simulink model "Psk"  (Simulink 8.9)
settings: Solver=ode45  StartTime=0.0  StopTime=100  RelTol=1e-3  EnableMultiTasking=on
libraries: commrandsrc2 x1, dsparch4 x1
settings Model: Creator=Abhishek  LastModifiedBy=JBlanco
settings DataIOCC: SignalLoggingSaveFormat=Dataset
settings DebuggingCC: SolverPrmCheckMsg=warning  FcnCallInpInsideContextMsg=error
settings GRTTargetCC: CombineOutputUpdateFcns=on  GRTInterface=off

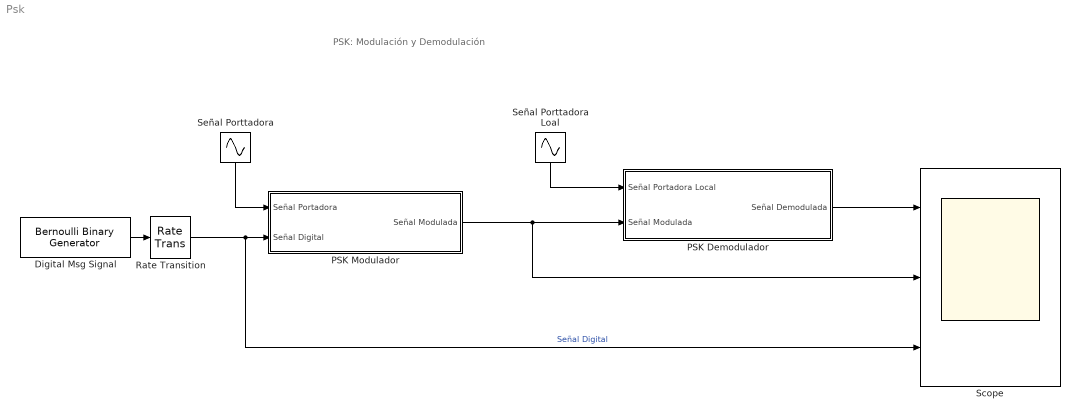
== system Psk ==
  note: PSK: Modulación y Demodulación
  Digital Msg Signal : commrandsrc2/Bernoulli Binary Generator  P=0.5  seed=61  Ts=5  frameBased=off  sampPerFrame=1  orient=off  outDataType=double  mask(Bernoulli Binary Generator){}
      mask Display:
      | % This is a new mask on top of the base mask.
      | % Use "View base mask" link below to see the base mask.
      | disp('Digital Data Gen.')
  PSK Demodulador : Subsystem
  PSK Modulador : Subsystem
  Rate Transition : RateTransition  OutPortSampleTime=1/2000
  Scope : Scope  NumInputPorts=3
  "Señal Porttadora " : Sin  Amplitude=5  Frequency=10*2*pi  Samples=50  SampleTime=1/2000
  Señal Porttadora Loal : Sin  Amplitude=5  Frequency=10*2*pi  Samples=50  SampleTime=1/2000
  wires:
  Digital Msg Signal/1 -> Rate Transition/1
  PSK Modulador/1(Señal Modulada) -> PSK Demodulador/2(Señal Modulada), Scope/2
  "Señal Porttadora "/1 -> PSK Modulador/1(Señal Portadora)
  Rate Transition/1 -> Scope/3, PSK Modulador/2(Señal Digital)  "Señal Digital"
  Señal Porttadora Loal/1 -> PSK Demodulador/1(Señal Portadora Local)
  PSK Demodulador/1(Señal Demodulada) -> Scope/1

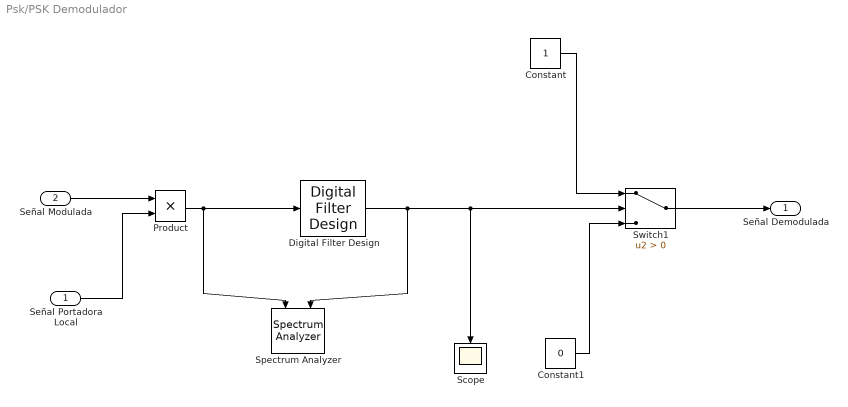
== system Psk/PSK Demodulador ==
  Señal Portadora Local : Inport
  Señal Modulada : Inport  Port=2
  Constant : Constant
  Constant1 : Constant  Value=0
  Digital Filter Design : dsparch4/Digital Filter Design  mwdsp_browser_bugfix_var=off
  Product : Product
  Scope : Scope
  Spectrum Analyzer : SpectrumAnalyzer  NumInputPorts=2
  Switch1 : Switch  Criteria=u2 > Threshold
  Señal Demodulada : Outport
  wires:
  Señal Modulada/1 -> Product/1
  Señal Portadora Local/1 -> Product/2
  Product/1 -> Digital Filter Design/1, Spectrum Analyzer/1
  Constant/1 -> Switch1/1
  Switch1/1 -> Señal Demodulada/1
  Constant1/1 -> Switch1/3
  Digital Filter Design/1 -> Spectrum Analyzer/2, Scope/1, Switch1/2

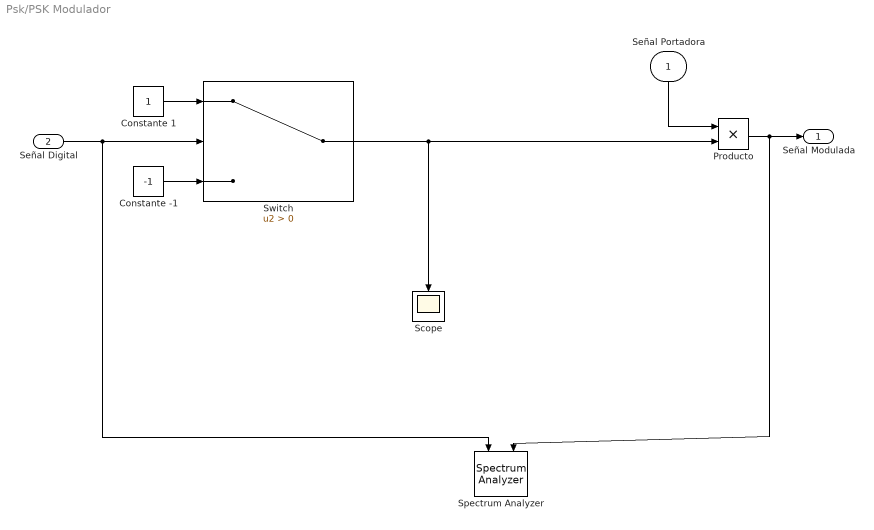
== system Psk/PSK Modulador ==
  Señal Portadora : Inport
  Señal Digital : Inport  Port=2
  Constante -1 : Constant  Value=-1
  Constante 1 : Constant
  Producto : Product
  Scope : Scope
  Spectrum Analyzer : SpectrumAnalyzer  NumInputPorts=2
  Switch : Switch  Criteria=u2 > Threshold
  Señal Modulada : Outport
  wires:
  Señal Digital/1 -> Spectrum Analyzer/1, Switch/2
  Constante -1/1 -> Switch/3
  Constante 1/1 -> Switch/1
  Switch/1 -> Scope/1, Producto/2
  Señal Portadora/1 -> Producto/1
  Producto/1 -> Spectrum Analyzer/2, Señal Modulada/1
